simulink model "motor_controller"  (R2019a)
settings: Solver=VariableStepAuto  StartTime=0.0  StopTime=50.0  RelTol=1e-3
libraries: arduinolib x8, simulink x2
settings Model: Creator=fotoyis  LastModifiedBy=fotoyis

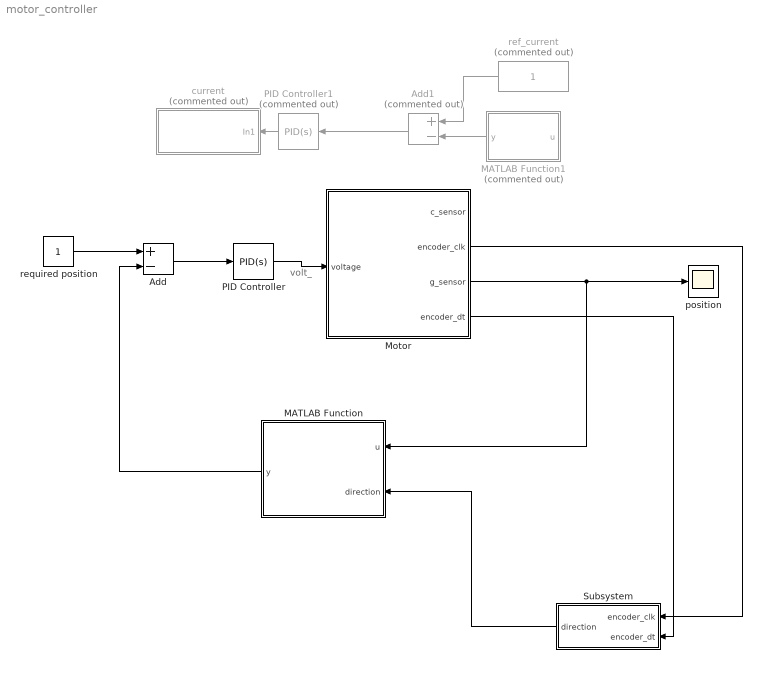
== system motor_controller ==
  note: volt_
  Add : Sum  Inputs=+-
  Add1 : Sum  Commented=on  Inputs=+-
  MATLAB Function : MATLAB Function  TreatAsAtomicUnit=on
  MATLAB Function1 : MATLAB Function  Commented=on  TreatAsAtomicUnit=on
  Motor : Subsystem
  PID Controller : simulink/Continuous/PID Controller  Controller=PID  Form=Parallel  TimeDomain=Continuous-time  SampleTime=-1  IntegratorMethod=Forward Euler  FilterMethod=Forward Euler  ControllerParametersSource=internal  P=1  I=1  D=0  UseFilter=on  N=100  TunerSelectOption=Transfer Function Based (PID Tuner App)  InitialConditionSource=internal  InitialConditionForIntegrator=0  InitialConditionForFilter=0  DifferentiatorICPrevScaledInput=0  ExternalReset=none  TrackingMode=off  Kt=1  LimitOutput=off  UpperSaturationLimit=inf  LowerSaturationLimit=-inf  LinearizeAsGain=on  AntiWindupMode=none  Kb=1  POutMin=[]  POutMax=[]  IOutMin=[]  IOutMax=[]  DOutMin=[]  DOutMax=[]  NOutMin=[]  NOutMax=[]  SumOutMin=[]  SumOutMax=[]  SaturationOutMin=[]  SaturationOutMax=[]  PParamMin=[]  PParamMax=[]  IParamMin=[]  IParamMax=[]  DParamMin=[]  DParamMax=[]  NParamMin=[]  NParamMax=[]  KbParamMin=[]  KbParamMax=[]  KtParamMin=[]  KtParamMax=[]  KbOutMin=[]  KbOutMax=[]  KtOutMin=[]  KtOutMax=[]  IntegratorOutMin=[]  IntegratorOutMax=[]  FilterOutMin=[]  FilterOutMax=[]  SumI1OutMin=[]  SumI1OutMax=[]  SumI2OutMin=[]  SumI2OutMax=[]  SumI3OutMin=[]  SumI3OutMax=[]  SumI4OutMin=[]  SumI4OutMax=[]  SumDOutMin=[]  SumDOutMax=[]  DifferentiatorOutMin=[]  DifferentiatorOutMax=[]  FilterDiffOutCoefMin=[]  FilterDiffOutCoefMax=[]  ReciprocalOutMin=[]  ReciprocalOutMax=[]  SumDenOutMin=[]  SumDenOutMax=[]  SumNumOutMin=[]  SumNumOutMax=[]  DivideOutMin=[]  DivideOutMax=[]  IntegratorContinuousStateAttributes=''  IntegratorStateMustResolveToSignalObject=off  IntegratorRTWStateStorageClass=Auto  FilterContinuousStateAttributes=''  FilterStateMustResolveToSignalObject=off  FilterRTWStateStorageClass=Auto  ParallelPVariant=InternalParameters  IdealPVariant=Disabled  IVariant=InternalParameters  DVariant=InternalParameters  IntegratorVariant=Continuous  SatVariant=Disabled  AWVariant=Passthrough  PCopyVariant=Disabled  TRVariant=Disabled  FdbkBlocksVariant=Forward  IdealPFdbkVariant=Disabled  SatFdbkVariant=Disabled  DerivativeFilterVariant=ContFilter  NVariant=InternalParameters  NCopyVariant=Disabled  FilterICVariant=InternalICsFilter  IntegratorICVariant=InternalICs  ExternalResetVariant=Disabled  TRSumVariant=Passthrough  SumFdbkVariant=Disabled  SumVariant=Sum_PID
  PID Controller1 : simulink/Continuous/PID Controller  Commented=on  Controller=PID  Form=Parallel  TimeDomain=Continuous-time  SampleTime=-1  IntegratorMethod=Forward Euler  FilterMethod=Forward Euler  ControllerParametersSource=internal  P=1  I=1  D=0  UseFilter=on  N=100  TunerSelectOption=Transfer Function Based (PID Tuner App)  InitialConditionSource=internal  InitialConditionForIntegrator=0  InitialConditionForFilter=0  DifferentiatorICPrevScaledInput=0  ExternalReset=none  TrackingMode=off  Kt=1  LimitOutput=off  UpperSaturationLimit=inf  LowerSaturationLimit=-inf  LinearizeAsGain=on  AntiWindupMode=none  Kb=1  POutMin=[]  POutMax=[]  IOutMin=[]  IOutMax=[]  DOutMin=[]  DOutMax=[]  NOutMin=[]  NOutMax=[]  SumOutMin=[]  SumOutMax=[]  SaturationOutMin=[]  SaturationOutMax=[]  PParamMin=[]  PParamMax=[]  IParamMin=[]  IParamMax=[]  DParamMin=[]  DParamMax=[]  NParamMin=[]  NParamMax=[]  KbParamMin=[]  KbParamMax=[]  KtParamMin=[]  KtParamMax=[]  KbOutMin=[]  KbOutMax=[]  KtOutMin=[]  KtOutMax=[]  IntegratorOutMin=[]  IntegratorOutMax=[]  FilterOutMin=[]  FilterOutMax=[]  SumI1OutMin=[]  SumI1OutMax=[]  SumI2OutMin=[]  SumI2OutMax=[]  SumI3OutMin=[]  SumI3OutMax=[]  SumI4OutMin=[]  SumI4OutMax=[]  SumDOutMin=[]  SumDOutMax=[]  DifferentiatorOutMin=[]  DifferentiatorOutMax=[]  FilterDiffOutCoefMin=[]  FilterDiffOutCoefMax=[]  ReciprocalOutMin=[]  ReciprocalOutMax=[]  SumDenOutMin=[]  SumDenOutMax=[]  SumNumOutMin=[]  SumNumOutMax=[]  DivideOutMin=[]  DivideOutMax=[]  IntegratorContinuousStateAttributes=''  IntegratorStateMustResolveToSignalObject=off  IntegratorRTWStateStorageClass=Auto  FilterContinuousStateAttributes=''  FilterStateMustResolveToSignalObject=off  FilterRTWStateStorageClass=Auto  ParallelPVariant=InternalParameters  IdealPVariant=Disabled  IVariant=InternalParameters  DVariant=InternalParameters  IntegratorVariant=Continuous  SatVariant=Disabled  AWVariant=Passthrough  PCopyVariant=Disabled  TRVariant=Disabled  FdbkBlocksVariant=Forward  IdealPFdbkVariant=Disabled  SatFdbkVariant=Disabled  DerivativeFilterVariant=ContFilter  NVariant=InternalParameters  NCopyVariant=Disabled  FilterICVariant=InternalICsFilter  IntegratorICVariant=InternalICs  ExternalResetVariant=Disabled  TRSumVariant=Passthrough  SumFdbkVariant=Disabled  SumVariant=Sum_PID
  Subsystem : Subsystem
  current : Subsystem  Commented=on
  position : Scope
  ref_current : Constant  Commented=on
  required position : Constant
  wires:
  required position/1 -> Add/1
  PID Controller/1 -> Motor/1(voltage)
  Add/1 -> PID Controller/1
  Motor/3(g_sensor) -> MATLAB Function/1(u), position/1
  MATLAB Function/1(y) -> Add/2
  MATLAB Function1/1(y) -> Add1/2
  Add1/1 -> PID Controller1/1
  PID Controller1/1 -> current/1(In1)
  ref_current/1 -> Add1/1
  Subsystem/1(direction) -> MATLAB Function/2(direction)
  Motor/2(encoder_clk) -> Subsystem/1(encoder_clk)
  Motor/4(encoder_dt) -> Subsystem/2(encoder_dt)

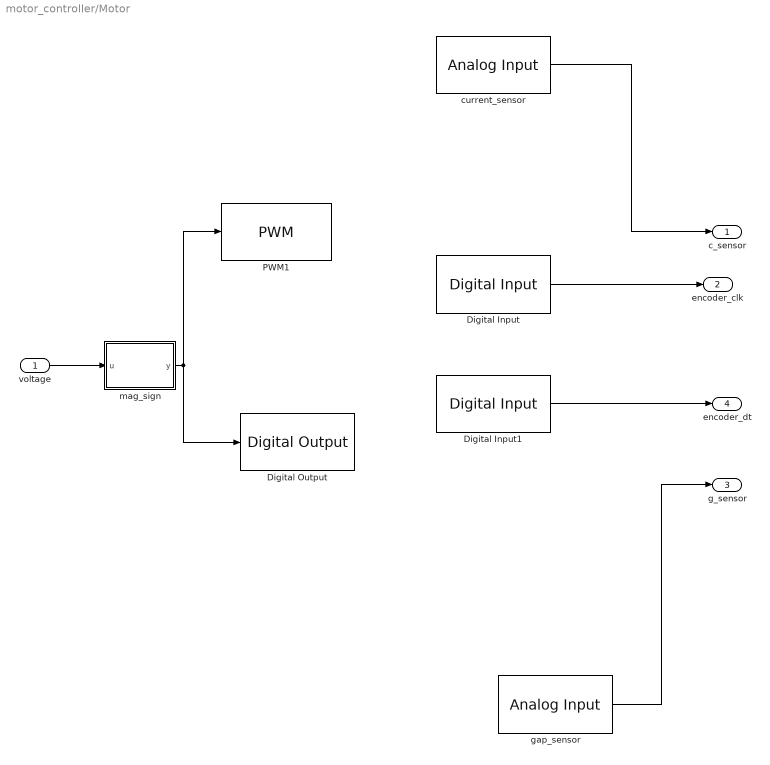
== system motor_controller/Motor ==
  voltage : Inport
  Digital Input : arduinolib/Digital Input  pinNumber=8  sampleTime=0.1  blockPlatform=arduino
      settings: SourceProductName=Simulink Support Package for Arduino Hardware
  Digital Input1 : arduinolib/Digital Input  pinNumber=8  sampleTime=0.1  blockPlatform=arduino
      settings: SourceProductName=Simulink Support Package for Arduino Hardware
  Digital Output : arduinolib/Digital Output  pinNumber=9  blockPlatform=arduino
  PWM1 : arduinolib/PWM  pinNumber=5  EnableInputFrequency=off  InitialFrequency=2000  InitialDutyCycle=0  NotificationType=None  blockPlatform=arduino
  current_sensor : arduinolib/Analog Input  pinNumber=4  ReadResultsOnly=off  ConversionTriggerSource=Software  ExternalTriggerType=uint32(0)  OutputDataType=uint16  EnableConversionCompleteNotify=off  EnableOuputStatus=off  SampleTime=1  blockPlatform=arduino
  gap_sensor : arduinolib/Analog Input  pinNumber=4  ReadResultsOnly=off  ConversionTriggerSource=Software  ExternalTriggerType=uint32(0)  OutputDataType=uint16  EnableConversionCompleteNotify=off  EnableOuputStatus=off  SampleTime=1  blockPlatform=arduino
  mag_sign : MATLAB Function  TreatAsAtomicUnit=on
  c_sensor : Outport
  encoder_clk : Outport  Port=2
  g_sensor : Outport  Port=3
  encoder_dt : Outport  Port=4
  wires:
  voltage/1 -> mag_sign/1(u)
  mag_sign/1(y) -> Digital Output/1, PWM1/1
  current_sensor/1 -> c_sensor/1
  Digital Input/1 -> encoder_clk/1
  gap_sensor/1 -> g_sensor/1
  Digital Input1/1 -> encoder_dt/1

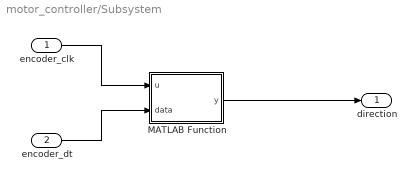
== system motor_controller/Subsystem ==
  encoder_clk : Inport
  encoder_dt : Inport  Port=2
  MATLAB Function : MATLAB Function  TreatAsAtomicUnit=on
  direction : Outport
  wires:
  encoder_clk/1 -> MATLAB Function/1(u)
  encoder_dt/1 -> MATLAB Function/2(data)
  MATLAB Function/1(y) -> direction/1

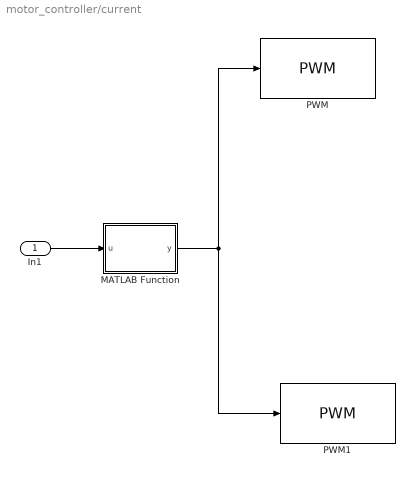
== system motor_controller/current ==
  In1 : Inport
  MATLAB Function : MATLAB Function  TreatAsAtomicUnit=on
  PWM : arduinolib/PWM  pinNumber=5  EnableInputFrequency=off  InitialFrequency=2000  InitialDutyCycle=0  NotificationType=None  blockPlatform=arduino
  PWM1 : arduinolib/PWM  pinNumber=5  EnableInputFrequency=off  InitialFrequency=2000  InitialDutyCycle=0  NotificationType=None  blockPlatform=arduino
  wires:
  In1/1 -> MATLAB Function/1(u)
  MATLAB Function/1(y) -> PWM/1, PWM1/1

== matlab function motor_controller/MATLAB Function ==
  data: u input; y output; direction input
function y = fcn(u, direction)

y = u;

== matlab function motor_controller/Motor/mag_sign ==
  data: u input; y output
function y = fcn(u)

y = u;

== matlab function motor_controller/MATLAB Function1 ==
  data: u input; y output
function y = fcn(u)

y = u;

== matlab function motor_controller/current/MATLAB Function ==
  data: u input; y output
function y = fcn(u)

y = u;

== matlab function motor_controller/Subsystem/MATLAB Function ==
  data: u input; y output; data input
function y = fcn(u, data)

y = u;
